simulink library "tenneco_lib"  (R2016b)
settings: Solver=ode45  StartTime=0.0  StopTime=10.0  RelTol=1e-3
undefined symbols (not defined in the file): Com_cntAMBInitTO_c, Com_cntAMBStopTO_c, Com_cntEC1InitTO_c, Com_cntEC1StopTO_c, Com_swAMBRx_c, Com_swEC1Rx_c, Com_swUseSPN108_c, Com_swUseSPN543_c, const, Env_pAmbPDflt_c, Env_pAmbPKOff_c, Env_pAmbPOvrd_c, Env_swAmbPOvrd_c, MSG_INIT_TIMEOUT, MSG_NOT_RECEIVED, MSG_RECEIVED_NOW, MSG_STOP_TIMEOUT
libraries: simulink x19, tenneco_lib x2
(part 1 of 5)
settings Model: Creator=artimahe  LastModifiedBy=jwd5048
settings Model: ModifiedComment=|
  | jwd5048 -- Fri Dec 14 12:11:19 2018 -- Version 1.13
  | 
  | Changed Rate Trasnition block info to have output sample time visible; Updated SWC template to have root level I/O; Subsyetem librart blocks (filters, timers etc) are set to run as Atomic
settings Model: ModifiedHistory=|
  | jwd5048 -- Fri Dec 14 12:11:19 2018 -- Version 1.13
  | 
  | Changed Rate Trasnition block info to have output sample time visible; Updated SWC template to have root level I/O; Subsyetem librart blocks (filters, timers etc) are set to run as Atomic
  | 
  | jwd5048 -- Sun Dec 09 17:40:26 2018 -- Version 1.12
  | 
  | Added report generator inport, outport, documentation blocks, Report Generator Subsystem, Updated LUTs for output data type in table data
settings DataIOCC: LimitDataPoints=on  SaveFormat=Array
settings OptimizationCC: BlockReduction=off  BooleanDataType=off  LifeSpan=inf
settings DebuggingCC: SaveWithParameterizedLinksMsg=none  UnderspecifiedInitializationDetection=Classic  MergeDetectMultiDrivingBlocksExec=none  SignalResolutionControl=TryResolveAllWithWarning  StrictBusMsg=Warning  SFUnexpectedBacktrackingDiag=warning  SFNoUnconditionalDefaultTransitionDiag=warning  SFExecutionAtInitializationDiag=none
settings HardwareCC: ProdBitPerPointer=32  ProdBitPerSizeT=32  ProdBitPerPtrDiffT=32  ProdLargestAtomicFloat=None  ProdIntDivRoundTo=Undefined  ProdEndianess=Unspecified  ProdWordSize=32  ProdHWDeviceType=32-bit Generic  TargetUnknown=on
settings ModelReferenceCC: PropagateSignalLabelsOutOfModel=off
settings GRTTargetCC: TargetLangStandard=C89/C90 (ANSI)  GeneratePreprocessorConditionals=Disable all
settings ConfigComp: CovMetricSettings=dw  CovHtmlReporting=on  CovSaveCumulativeToWorkspaceVar=on  CovSaveSingleToWorkspaceVar=on  CovExternalEMLEnable=off  CovSFcnEnable=off

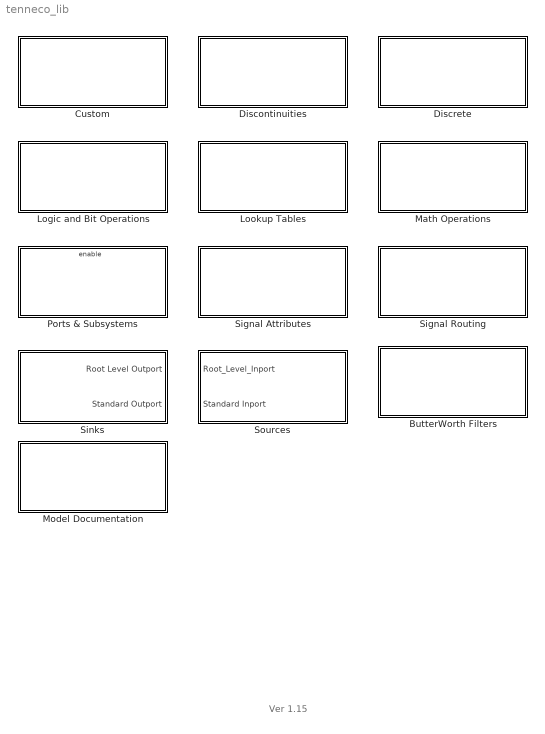
== system tenneco_lib ==
  note: Ver 1.15
  ButterWorth Filters : Subsystem
      mask Display: disp('Filters');
  Custom : Subsystem
      mask Display: disp('Custom');
  Discontinuities : Subsystem
      mask Display: disp('Discontinuities');
  Discrete : Subsystem
      mask Display: disp('Discrete');
  Logic and Bit Operations : Subsystem
      mask Display: disp('Logic and Bit Operations');
  Lookup Tables : Subsystem
      mask Display: disp('Lookup Tables');
  Math Operations : Subsystem
      mask Display: disp('Math Operations');
  Model Documentation : Subsystem
      mask Display: disp('Model Documentation');
  Ports & Subsystems : Subsystem
      mask Display: disp('Ports & Subsystems');
  Signal Attributes : Subsystem
      mask Display: disp('Signal Attributes');
  Signal Routing : Subsystem
      mask Display: disp('Signal Routing');
  Sinks : Subsystem
      mask Display: disp('Sinks');
  Sources : Subsystem
      mask Display: disp('Sources');

== system tenneco_lib/ButterWorth Filters ==
  Butterworth First Order HPF : Subsystem  TreatAsAtomicUnit=on  mask(Filter){Ts=.001}
      mask prompts: Ts "sample time(sec)"
      mask help: Butterworth First Order HPF
      mask Display:
      | image(imread('Tenneco_Copyright_Logo_Mini.bmp'),'center');
      | color('red');
      | disp('\n\n\n\n\n\n\nTenneco Confidential Red\n Restricted. Do not Distribute.');
  Butterworth First Order LPF : Subsystem  TreatAsAtomicUnit=on  mask(Filter){Ts=.001}
      mask prompts: Ts "sample time(sec)"
      mask help: Butterworth First Order LPF
      mask Display:
      | image(imread('Tenneco_Copyright_Logo_Mini.bmp'),'center');
      | color('red');
      | disp('\n\n\n\n\n\n\nTenneco Confidential Red\n Restricted. Do not Distribute.');
  Butterworth Second Order BPF : Subsystem  TreatAsAtomicUnit=on  mask(Filter){Ts=0.001}
      mask prompts: Ts "sample time(sec)"
      mask help: Butterworth Second Order BPF
      mask Display:
      | image(imread('Tenneco_Copyright_Logo_Mini.bmp'),'center');
      | color('red');
      | disp('\n\n\n\n\n\n\nTenneco Confidential Red\n Restricted. Do not Distribute.');
  Butterworth Second Order HPF : Subsystem  TreatAsAtomicUnit=on  mask(Filter){Ts=.001}
      mask prompts: Ts "sample time(sec)"
      mask help: Butterworth Second Order HPF
      mask Display:
      | image(imread('Tenneco_Copyright_Logo_Mini.bmp'),'center');
      | color('red');
      | disp('\n\n\n\n\n\n\nTenneco Confidential Red\n Restricted. Do not Distribute.');
  Butterworth Second Order LPF : Subsystem  TreatAsAtomicUnit=on  mask(Filter){Ts=.001}
      mask prompts: Ts "sample time(sec)"
      mask help: Butterworth Second Order LPF
      mask Display:
      | image(imread('Tenneco_Copyright_Logo_Mini.bmp'),'center');
      | color('red');
      | disp('\n\n\n\n\n\n\nTenneco Confidential Red\n Restricted. Do not Distribute.');
  Generic Low-Pass Filter : Subsystem  TreatAsAtomicUnit=on  mask{Fil=.01, SampleTime=1, N=2}
      mask prompts: Fil "Filter Coefficient"; SampleTime "Sample Time in Seconds"; N "Stabilization Time [# loops]"
      mask help:
      | Filter coefficient=sampletime/number of samples to be averaged
      | Please use explicit sample time. Do not use (-1).
      |
      | The initial condition of the filter will be the input value after the
      | stabilization period has expired.
      mask Display:
      | port_label('input',1,'x');
      | port_label('output',1,'y');
      | 
      | image(imread('Tenneco_Copyright_Logo_Mini.bmp'),'center');
      | color('red');
      | disp('\n\n\n\n\n\n\nTenneco Confidential Red\n Restricted. Do not Distribute.');
  Resettable Variable Low-Pass Filter : Subsystem  TreatAsAtomicUnit=on  mask{Ts=0.1, N=2}
      mask prompts: Ts "Filter Sample Time [sec]"; N "Stabilization Loops [#]"
      mask help:
      | The initial condition of the filter will be the input value after the
      | stabilization period has expired.
      mask init:
      | if (isempty(N) || ...
      |         rem(N, 1) ~= 0 || ...
      |        (rem(N, 1) == 0 && N < 1))
      |         errordlg(['Number of stabilization loops must be a ' ...
      |                  'positive integer.'], ...
      |                  'Error: Function Block Parameters');
      | end
      | 
      | if (isempty(Ts) || ...
      |         (Ts <= 0))
      |         errordlg(['Sample time must be greater than zero.'], ...
      |                  'Error: Function Block Parameters');
      | end
      mask Display:
      | port_label('input',1,'x');
      | port_label('input',2,'t [sec]');
      | port_label('input',3,'reset');
      | port_label('output',1,'y');
      | 
      | image(imread('Tenneco_Copyright_Logo_Mini.bmp'),'center');
      | color('red');
      | disp('\n\n\n\n\n\n\nTenneco Confidential Red\n Restricted. Do not Distribute.');
  Variable Low-Pass Filter : Subsystem  TreatAsAtomicUnit=on  mask{Ts=0.1, N=2}
      mask prompts: Ts "Filter Sample Time [sec]"; N "Stabilization Loops [#]"
      mask help:
      | The initial condition of the filter will be the input value after the
      | stabilization period has expired.
      mask init: same as tenneco_lib/ButterWorth Filters/Resettable Variable Low-Pass Filter
      mask Display:
      | port_label('input',1,'x');
      | port_label('input',2,'\tau [sec]','texmode','on');
      | port_label('output',1,'y');
      | 
      | image(imread('Tenneco_Copyright_Logo_Mini.bmp'),'center');
      | color('red');
      | disp('\n\n\n\n\n\n\nTenneco Confidential Red\n Restricted. Do not Distribute.');

== system tenneco_lib/Custom ==
  CAN : Subsystem
      mask Display: disp('CAN');
  Logical : Subsystem
      mask Display: disp('Logical');
  Math : Subsystem
      mask Display: disp('Math');
  Timers : Subsystem
      mask Display: disp('Timers');

== system tenneco_lib/Discontinuities ==
  Rate Limiter Dynamic : simulink/Discontinuities/Rate Limiter Dynamic
  Saturation : Saturate  UpperLimit=UpperLimit  LowerLimit=LowerLimit  mask(Saturation){UpperLimit=0.5, LowerLimit=-0.5}
      mask prompts: UpperLimit "Simulink:blkprm_prompts:SaturateUpLim"; LowerLimit "Simulink:blkprm_prompts:SaturateLowLim"
      mask help: Limit input signal to the upper and lower saturation values.
      settings: CopyFcn=set_param(gcbh,'LinkStatus','none');
      mask TypeOptions UpperLimit: UpperLimit
      mask TypeOptions LowerLimit: LowerLimit

== system tenneco_lib/Discrete ==
  Discrete Filter : DiscreteFilter  NumeratorSource=Input port  DenominatorSource=Input port  a0EqualsOne=on  mask(Discrete Filter){}
      mask help: Independently filter each channel of the input over time using a discrete IIR filter. Specify the numerator and denominator coefficients in ascending order of powers of 1/z.
      settings: CopyFcn=set_param(gcbh,'LinkStatus','none');  InputPortMap=u0,p1,p3
  Unit Delay : UnitDelay  InitialCondition=InitialCondition  SampleTime=-1  mask(Unit Delay){InitialCondition=0}
      mask prompts: InitialCondition "Simulink:blkprm_prompts:DelayBlkInitCond"
      mask help: Sample and hold with one sample period delay.
      settings: CopyFcn=set_param(gcbh,'LinkStatus','none');
      mask TypeOptions InitialCondition: InitialCondition

== system tenneco_lib/Logic and Bit Operations ==
  Bitwise Operator : simulink/Logic and Bit Operations/Bitwise Operator  logicop=AND  UseBitMask=on  BitMask=bin2dec('11011001')  BitMaskRealWorld=Stored Integer
  Compare To Constant : simulink/Logic and Bit Operations/Compare To Constant  relop=<=  const=const  OutDataTypeStr=boolean
  Logical Operator : Logic  Inputs=Inputs  AllPortsSameDT=off  OutDataTypeStr=boolean  mask(Logical Operator){Operator=AND, Inputs=2}
      mask prompts: Operator "Simulink:blkprm_prompts:LogicOperator"; Inputs "Simulink:blkprm_prompts:LogicNumInputPorts"
      mask help: Logical operators. For a single input, operators are applied across the input vector. For multiple inputs, operators are applied across the inputs.
      settings: CopyFcn=set_param(gcbh,'LinkStatus','none');
      mask TypeOptions Operator: Operator
      mask TypeOptions Inputs: Inputs
  Relational Operator : RelationalOperator  Operator=<=  OutDataTypeStr=boolean  RndMeth=Nearest  mask(Relational Operator){Operator=<=}
      mask prompts: Operator "Simulink:blkprm_prompts:RelopOperator"
      mask help: Applies the selected relational operator to the inputs and outputs the result. The top (or left) input corresponds to the first operand.
      settings: CopyFcn=set_param(gcbh,'LinkStatus','none');
      mask TypeOptions Operator: Operator
  Shift Arithmetic : ArithShift  BitShiftNumber=8
      settings: CopyFcn=set_param(gcbh,'LinkStatus','none');

== system tenneco_lib/Lookup Tables ==
  1-D Lookup Table : Lookup_n-D  NumberOfTableDimensions=1  BreakpointsForDimension1=BreakpointsForDimension1  BreakpointsForDimension3=[5, 7]  Table=Table  ExtrapMethod=Clip  UseLastTableValue=on  InternalRulePriority=Speed  OutDataTypeStr=Inherit: Inherit from 'Table data'  RndMeth=Simplest  LockScale=on  mask(Lookup Table (1-D)){Table=[1,2,3], BreakpointsForDimension1=[10,22,31]}
      mask prompts: Table "Simulink:blkprm_prompts:InterpndTable"; BreakpointsForDimension1 "Breakpoints for axis:"
      mask help: Perform 1-dimensional interpolated table lookup including index searches. The table is a sampled representation of a function in N variables. Breakpoint sets relate the input values to positions in the table.
      settings: CopyFcn=set_param(gcbh,'LinkStatus','none');
      mask TypeOptions Table: Table
      mask TypeOptions BreakpointsForDimension1: BreakpointsForDimension1
  2-D Lookup Table : Lookup_n-D  BreakpointsForDimension1=BreakpointsForDimension1  BreakpointsForDimension2=BreakpointsForDimension2  BreakpointsForDimension3=[5, 7]  Table=Table  ExtrapMethod=Clip  UseLastTableValue=on  InternalRulePriority=Speed  OutDataTypeStr=Inherit: Inherit from 'Table data'  RndMeth=Simplest  LockScale=on  mask(Lookup Table (2-D)){Table=[1,2,3;4,5,6], BreakpointsForDimension1=[10,22], BreakpointsForDimension2=[10,22,31]}
      mask prompts: Table "Simulink:blkprm_prompts:InterpndTable"; BreakpointsForDimension1 "Breakpoints for u1 (y-axis):"; BreakpointsForDimension2 "Breakpoints for u2 (x-axis):"
      mask help: Perform 2-dimensional interpolated table lookup including index searches. The table is a sampled representation of a function in N variables. Breakpoint sets relate the input values to positions in the table. The first dimension corresponds to the top (or left) input port.
      settings: CopyFcn=set_param(gcbh,'LinkStatus','none');
      mask TypeOptions Table: Table
      mask TypeOptions BreakpointsForDimension1: BreakpointsForDimension1
      mask TypeOptions BreakpointsForDimension2: BreakpointsForDimension2

== system tenneco_lib/Math Operations ==
  Abs : Abs  mask(Abs){}
      mask help: y = |u|
      settings: CopyFcn=set_param(gcbh,'LinkStatus','none');
  Gain : Gain  Gain=Gain  mask(Gain){Gain=1}
      mask prompts: Gain "Simulink:blkprm_prompts:GainGain"
      mask help: Element-wise gain (y = K.*u) or matrix gain (y = K*u or y = u*K).
      mask init:
      | blkName = gcb;
      | 
      | str = ['C']; %default
      | 
      | const_str = get_param(blkName, 'Gain');
      | const_val = str2num(const_str);
      | 
      | if isempty(const_val) %#ok<ST2NM>
      |     %Expression/Variable
      |     str = [strtrim(const_str)];
      | else
      |     if length(const_val) == 1 
      |         if Simulink.data.isSupportedEnumClass(class(const_val))
      |             % Special Handling for Enumerations
      |             if Simulink.data.getEnumTypeInfo(class(const_val), 'AddClassNameToEnumNames')
      |                 str = [strtrim(const_str)];
      |             else
      |                 str = [char(const_val)];
      |             end
      |         elseif(isfloat(const_val) || isinteger(const_val)) 
      |                 str = [num2str(const_val)];
      |         end
      |     end
      | end
      settings: CopyFcn=set_param(gcbh,'LinkStatus','none');
      mask TypeOptions Gain: Gain
      mask Display: disp(strcat('GAIN\n',str))
  Math Function : Math  Operator=square  SaturateOnIntegerOverflow=on  mask(Math){Operator=square}
      mask prompts: Operator "SimulinkBlocks:dialog:BmathfcnOperator"
      mask help: Mathematical functions including logarithmic, exponential, power, and modulus functions. When the function has more than one argument, the first argument corresponds to the top (or left) input port.
      settings: CopyFcn=set_param(gcbh,'LinkStatus','none');
      mask TypeOptions Operator: Operator
  MinMax : MinMax  Inputs=Inputs  mask(MinMax){Function=min, Inputs=1}
      mask prompts: Function "Simulink:blkprm_prompts:MinMaxFunction"; Inputs "Simulink:blkprm_prompts:MinMaxNumInPorts"
      mask help: Output min or max of input. For a single input, operators are applied across the input vector. For multiple inputs, operators are applied across the inputs.
      settings: CopyFcn=set_param(gcbh,'LinkStatus','none');
      mask TypeOptions Function: Function
      mask TypeOptions Inputs: Inputs
  Product : Product  Inputs=*/  InputSameDT=on  mask(Product){Inputs=*/}
      mask prompts: Inputs "List of signs:"
      mask help:
      | Multiply or divide inputs.  Specify one of the following:
      |  a) * or / for each input port. For example, **/* performs the operation 'u1*u2/u3*u4'.
      |  b) scalar specifies the number of input ports to be multiplied.
      settings: CopyFcn=set_param(gcbh,'LinkStatus','none');
      mask TypeOptions Inputs: Inputs
  Rounding Function : Rounding  Operator=round  mask(Rounding){Operator=round}
      mask prompts: Operator "Simulink:blkprm_prompts:RoundOperator"
      mask help: Rounding operations.
      settings: CopyFcn=set_param(gcbh,'LinkStatus','none');
      mask TypeOptions Operator: Operator
  Sqrt : Sqrt  SaturateOnIntegerOverflow=on  mask(Sqrt){Operator=sqrt}
      mask prompts: Operator "SimulinkBlocks:SqrtFcn:BmathfcnOperator"
      mask help: Square root functions including square root, signed square root, and reciprocal square root functions.
      settings: CopyFcn=set_param(gcbh,'LinkStatus','none');
      mask TypeOptions Operator: Operator
  Sum : Sum  Inputs=+-  InputSameDT=on  mask(Sum){Inputs=+-}
      mask prompts: Inputs "Simulink:blkprm_prompts:SumListofSigns"
      mask help:
      | Add or subtract inputs.  Specify one of the following:
      | a) character vector containing + or - for each input port, | for spacer between ports (e.g. ++|-|++)
      | b) scalar, >= 1, specifies the number of input ports to be summed.
      | When there is only one input port, add or subtract elements over all dimensions or one specified dimension
      settings: CopyFcn=set_param(gcbh,'LinkStatus','none');
      mask TypeOptions Inputs: Inputs
  Trigonometric Function : Trigonometry  mask(Trigonometric Function){Operator=sin}
      mask prompts: Operator "Simulink:blkprm_prompts:TrigFcnOperator"
      mask help: Trigonometric and hyperbolic functions. When the function has more than one argument, the first argument corresponds to the top (or left) input port.
      settings: CopyFcn=set_param(gcbh,'LinkStatus','none');
      mask TypeOptions Operator: Operator
  Unary Minus : UnaryMinus
      settings: CopyFcn=set_param(gcbh,'LinkStatus','none');

== system tenneco_lib/Model Documentation ==
  Appendix Title : Subsystem  mask(RptGen Appendix){rptgenOrder=10}
      mask prompts: rptgenOrder "Report Gen Order Priority"
      mask help:
      | This block is designed to contain RptGen Description and RptGen Detail blocks to create a document structure as an appendix to be added at the end of the MBDD.
      |
      | If this block is anywhere in a model, an appendix with the block name as the section title shall appear in the report.
      |
      | The Report Gen Order Priority allows the user to set the sorted order of the block's contents appearing in the report.
      settings: OpenFcn=open_system(gcb,'force')
      mask Display: disp(['Appendix - ',get_param(gcb,'rptgenOrder')])
  Description : Subsystem  mask(RptGenDescription){rptgenOrder=10}
      mask prompts: rptgenOrder "Report Gen Order Priority"
      mask help:
      | This block can contain text, tables, lists, images, and equations from a Word document to describe its parent subsystem.
      |
      | The contents of this block shall be placed in paragraph(s) just after the subsystem's section heading in the report, before the system snapshot.
      |
      | The Report Gen Order Priority allows the user to set the sorted order of the block's contents appearing in the report.
      settings: OpenFcn=open_system([gcb,'/DocBlock'])
      mask Display: disp(['Description - ',get_param(gcb,'rptgenOrder')])
  Detail : Subsystem  mask(RptGenDetail){rptgenOrder=10}
      mask prompts: rptgenOrder "Report Gen Order Priority"
      mask help:
      | This block can contain text, tables, lists, images, and equations from a Word document to further describe its parent subsystem, when a brief description is not sufficient to fully describe a system.
      |
      | The name of this block shall appear as the subsection title underneath the current subsystem's section.
      |
      | The Report Gen Order Priority allows the user to set the sorted order of the block's contents appearing in the report.
      settings: OpenFcn=open_system([gcb,'/DocBlock'])
      mask Display: disp(['Detail - ',get_param(gcb,'rptgenOrder')])
  Introduction : Subsystem  mask(RptGenIntroduction){rptgenOrder=10}
      mask prompts: rptgenOrder "Report Gen Order Priority"
      mask help:
      | This block can contain text, tables, lists, images, and equations from a Word document for the introduction portion of the MBDD.
      |
      | The contents of this block shall be placed in the introductory section if it is in a software part model.
      |
      | The Report Gen Order Priority allows the user to set the sorted order of the block's contents appearing in the report.
      settings: OpenFcn=open_system([gcb,'/DocBlock'])
      mask Display: disp(['Introduction - ',get_param(gcb,'rptgenOrder')])

== system tenneco_lib/Ports & Subsystems ==
  Enable : EnablePort  mask(Enable Port){StatesWhenEnabling=held, ShowOutputPort=off}
      mask prompts: StatesWhenEnabling "Simulink:blkprm_prompts:EnabPortStates"; ShowOutputPort "Simulink:blkprm_prompts:TrigEnabShowOutPort"
      mask help: Place this block in a subsystem or at the root level of a model to create an enabled system.
      settings: CopyFcn=set_param(gcbh,'LinkStatus','none');
      mask TypeOptions StatesWhenEnabling: StatesWhenEnabling
      mask TypeOptions ShowOutputPort: ShowOutputPort
  If : If  mask(If Block){NumInputs=1, IfExpression=u1 > 0, ElseIfExpressions=, ShowElse=on}
      mask prompts: NumInputs "Simulink:blkprm_prompts:IfNumInputs"; IfExpression "Simulink:blkprm_prompts:IfCondition"; ElseIfExpressions "Simulink:blkprm_prompts:ElseIfConds"; ShowElse "Simulink:blkprm_prompts:IfShowElse"
      mask help:
      | IF expression
      |     Run the Action Subsystem connected to 1st output port
      | ELSEIF expression
      |     Run the Action Subsystem connected to 2nd output port
      | ELSE
      |     Run the Action Subsystem connected to last output port
      | END
      | The number of Elseif output ports in the block is equal to the
      | number of comma-separated Elseif expressions entered in the dialog.
      | The If and Elseif expressions can use these MATLAB operators:
      |     <, <=, ==, ~=, >, >=, &, |, ~, (  ), unary-minus
      | on the input port signals named u1, u2, u3, etc.
      settings: CopyFcn=set_param(gcbh,'LinkStatus','none');
      mask TypeOptions NumInputs: NumInputs
      mask TypeOptions IfExpression: IfExpression
      mask TypeOptions ElseIfExpressions: ElseIfExpressions
      mask TypeOptions ShowElse: ShowElse
  If Action Subsystem : Subsystem  TreatAsAtomicUnit=on
      settings: CopyFcn=set_param(gcbh,'LinkStatus','none'); set_param(gcbh,'Mask','off'); set_param(gcbh,'MaskType',''); set_param(gcbh,'MaskDescription',''); set_param(gcbh,'OpenFcn',''); set_param(gcbh,'CopyFcn','')  OpenFcn=open_system(gcbh,'force')
  SoftwareComponent SWC : Subsystem  Tag=SoftwareComponent  mask(Software Component Subsystem){libVer=1.13, DataDictionary=SoftwareComponent_dd.m, swDescription=, logEntry=|}
      mask logEntry=|
      | jwd5048 -- Fri Dec 14 12:11:19 2018 -- Version 1.13
      |
      | Changed Rate Trasnition block info to have output sample time visible; Updated SWC template to have root level I/O; Subsyetem librart blocks (filters, timers etc) are set to run as Atomic
      mask prompts: libVer "Library Version"; DataDictionary "Data Dictionary File"; swDescription "Software Description"; logEntry "Version Log"
      mask help: Keeps track of the version of the software component and the corresponding data dictionary. Also contains an abstract description of the software component and the last version log entry.
      settings: PreSaveFcn=updateSwcParams  OpenFcn=open_system(gcb,'force')
      mask Help: If this subsystem resides inside the top layer of a Simulink diagram, changing the version number in the parameters pane will kick-off operations to update the model history and version number.  It will also run checks to make sure the log entry was updated and the version number was incremented properly, before pushing this information to the model parameters.
      mask DialogControl Control3 Prompt: Library Version:  %<libVer>
      mask DialogControl Container3 Prompt: Software Description
      mask DialogControl Control4 Prompt: %<swDescription>
      mask DialogControl Container4 Prompt: Version Log Entry
      mask DialogControl Control5 Prompt: %<logEntry>
      mask Display: disp(['Library Ver. ', get_param(gcb,'libVer'), '\nDD File: ', get_param(gcb,'DataDictionary')]);
  wires:
  If/1 -> If Action Subsystem/Action

== system tenneco_lib/Signal Attributes ==
  Data Type Conversion : DataTypeConversion  mask(Data Type Conversion){OutDataTypeStr=Inherit: Inherit via back propagation}
      mask prompts: OutDataTypeStr "Simulink:blkprm_prompts:OUTPUT_UNIFIEDDATATYPE"
      mask help: Convert the input to the data type and scaling of the output.
      settings: CopyFcn=set_param(gcbh,'LinkStatus','none');
      mask TypeOptions OutDataTypeStr: OutDataTypeStr
  Rate Transition : RateTransition
      settings: AttributesFormatString=%<OutPortSampleTime>  CopyFcn=set_param(gcbh,'LinkStatus','none');

== system tenneco_lib/Signal Routing ==
  Bus Creator : BusCreator  Inputs=2
      settings: CopyFcn=set_param(gcbh,'LinkStatus','none');
  Bus Selector : BusSelector  OutputSignals=signal1,signal2
      settings: CopyFcn=set_param(gcbh,'LinkStatus','none');
  Data Store Memory : DataStoreMemory  ReadBeforeWriteMsg=warning  WriteAfterWriteMsg=warning  WriteAfterReadMsg=warning  InitialValue=InitialValue  ShowAdditionalParam=off  mask(Data Store Memory){DataStoreName=A, InitialValue=0, OutDataTypeStr=Inherit: auto, Dimensions=-1}
      mask prompts: DataStoreName "Simulink:blkprm_prompts:DstoreMemDstoreName"; InitialValue "Simulink:blkprm_prompts:DstoreMemInitvalue"; OutDataTypeStr "Simulink:blkprm_prompts:UNIFIEDDATATYPE"; Dimensions "Simulink:blkprm_prompts:DstoreMemDimensions"
      mask help: Define a memory region for use by the Data Store Read and Data Store Write blocks. All Read and Write blocks that are in the current (sub)system level or below and have the same data store name will be able to read from or write to this block.
      settings: CopyFcn=set_param(gcbh,'LinkStatus','none');
      mask TypeOptions DataStoreName: DataStoreName
      mask TypeOptions InitialValue: InitialValue
      mask TypeOptions OutDataTypeStr: OutDataTypeStr
      mask TypeOptions Dimensions: Dimensions
  Data Store Read : DataStoreRead  SampleTime=SampleTime  mask(Data Store Read){DataStoreName=A, SampleTime=-1}
      mask prompts: DataStoreName "Simulink:blkprm_prompts:DstoreMemDstoreName"; SampleTime "Simulink:blkprm_prompts:AllSrcBlksSampleTime"
      mask help: Read values from the specified data store.
      settings: CopyFcn=set_param(gcbh,'LinkStatus','none');
      mask TypeOptions DataStoreName: DataStoreName
      mask TypeOptions SampleTime: SampleTime
  Data Store Write : DataStoreWrite  mask(Data Store Write){DataStoreName=A}
      mask prompts: DataStoreName "Simulink:blkprm_prompts:DstoreMemDstoreName"
      mask help: Write values to the specified data store.
      settings: CopyFcn=set_param(gcbh,'LinkStatus','none');
      mask TypeOptions DataStoreName: DataStoreName
  Demux : Demux  Outputs=2  mask(Demux){Outputs=2}
      mask prompts: Outputs "Simulink:blkprm_prompts:DemuxNumOfOutputs"
      mask help: Split vector signals into scalars or smaller vectors.
      settings: CopyFcn=set_param(gcbh,'LinkStatus','none');
      mask TypeOptions Outputs: Outputs
  Merge : Merge  Inputs=Inputs  InitialOutput=InitialOutput  mask(Merge){Inputs=2, InitialOutput=[]}
      mask prompts: Inputs "Simulink:blkprm_prompts:MergeNumInputs"; InitialOutput "Simulink:blkprm_prompts:MergeInitOutput"
      mask help: Merge the input signals into a single output signal whose initial value is specified by the 'Initial output' parameter. If 'Initial output' is empty, the Merge block outputs the initial output of one of its driving blocks.
      settings: CopyFcn=set_param(gcbh,'LinkStatus','none');
      mask TypeOptions Inputs: Inputs
      mask TypeOptions InitialOutput: InitialOutput
  Multiport Switch : MultiPortSwitch  DataPortOrder=Specify indices  DataPortIndices=DataPortIndices  DiagnosticForDefault=Warning  mask(Multiport Switch){DataPortIndices={1,2,3}}
      mask prompts: DataPortIndices "Simulink:blkprm_prompts:MpSwitch_DataPortIndices"
      mask help: Pass through the input signals corresponding to the truncated value of the first input. The inputs are numbered top to bottom (or left to right). The first input port is the control port. The other input ports are data ports.
      settings: CopyFcn=set_param(gcbh,'LinkStatus','none');
      mask TypeOptions DataPortIndices: DataPortIndices
  Mux : Mux  Inputs=2  mask(Mux){Inputs=2}
      mask prompts: Inputs "Simulink:blkprm_prompts:MuxNumInputs"
      mask help: Multiplex scalar or vector signals.
      settings: CopyFcn=set_param(gcbh,'LinkStatus','none');
      mask TypeOptions Inputs: Inputs
  Selector : Selector  IndexMode=Zero-based  InputPortWidth=3  IndexOptions=Index vector (dialog)  Indices=[1]  OutputSizes=1
      settings: CopyFcn=set_param(gcbh,'LinkStatus','none');
  Switch : Switch  Threshold=0.5  mask(Switch){}
      mask help: Pass through input 1 when input 2 satisfies the selected criterion; otherwise, pass through input 3. The inputs are numbered top to bottom (or left to right). The first and third input ports are data ports, and the second input port is the control port. The criteria for control port 2 are u2 >= Threshold (0.5).
      settings: CopyFcn=set_param(gcbh,'LinkStatus','none');
  Vector Concatenate : Concatenate  NumInputs=NumInputs  mask(Concatenate){NumInputs=2}
      mask prompts: NumInputs "Simulink:blkprm_prompts:ConcatNumInputs"
      mask help:
      | Concatenate input signals of the same data type to create a contiguous output signal.
      |
      | In vector mode, all input signals must be either vectors or one-row [1xM] matrices or one-column [Mx1] matrices or a combination of vectors and either one-row matrices or one-column matrices. The output is a vector if all inputs are vectors. The output is a one-row or one-column matrix if any of the inputs are one-row or one-column matrices, respectively.
      settings: CopyFcn=set_param(gcbh,'LinkStatus','none');
      mask TypeOptions NumInputs: NumInputs

== system tenneco_lib/Sinks ==
  Terminator : Terminator
      settings: CopyFcn=set_param(gcbh,'LinkStatus','none');
  Root Level Outport : Outport  OutMin=OutMin  OutMax=OutMax  SampleTime=SampleTime  mask(Root Level Outport){Port=1, OutDataTypeStr=Inherit: auto, PortDimensions=-1, SampleTime=-1, OutMin=[], OutMax=[], Unit=inherit}
      mask prompts: Port "Simulink:blkprm_prompts:InOutportPortNum"; OutDataTypeStr "Simulink:blkprm_prompts:UNIFIEDDATATYPE"; PortDimensions "Simulink:blkprm_prompts:InportPortDims"; SampleTime "Simulink:blkprm_prompts:AllBlksSampleTime"; OutMin "Simulink:blkprm_prompts:DesignMin"; OutMax "Simulink:blkprm_prompts:DesignMax"; Unit "Simulink:blkprm_prompts:OutputUnit_EditField"
      mask help: Provide a root level output port for a model.
      settings: CopyFcn=set_param(gcbh,'LinkStatus','none');
      mask TypeOptions Port: Port
      mask TypeOptions OutDataTypeStr: OutDataTypeStr
      mask TypeOptions PortDimensions: PortDimensions
      mask TypeOptions SampleTime: SampleTime
      mask TypeOptions OutMin: OutMin
      mask TypeOptions OutMax: OutMax
      mask TypeOptions Unit: Unit
  Standard Outport : Outport  Port=2  mask(Standard Outport){Port=2}
      mask prompts: Port "Simulink:blkprm_prompts:InOutportPortNum"
      mask help: Provide an output port for subsystems.
      settings: CopyFcn=set_param(gcbh,'LinkStatus','none');
      mask TypeOptions Port: Port

== system tenneco_lib/Sources ==
  Root_Level_Inport : Inport  OutMin=OutMin  OutMax=OutMax  Unit=m/s  PortDimensions=1  SampleTime=SampleTime  mask(Root Level Inport){Port=1, OutDataTypeStr=Inherit: auto, PortDimensions=1, Resolution=0.001, OutMin=-10, OutMax=10, Unit=m/s, SampleTime=-1, varSource=SoftwarePart_dd}
      mask prompts: Port "Simulink:blkprm_prompts:InOutportPortNum"; OutDataTypeStr "Simulink:blkprm_prompts:UNIFIEDDATATYPE"; PortDimensions "Simulink:blkprm_prompts:InportPortDims"; OutMin "Simulink:blkprm_prompts:DesignMin"; OutMax "Simulink:blkprm_prompts:DesignMax"; Unit "Simulink:blkprm_prompts:OutputUnit_EditField"; SampleTime "Simulink:blkprm_prompts:AllBlksSampleTime"; varSource "Signal Source"
      mask help:
      | Provide an input port for a software component.
      |
      | The data type, dimensions, and engineering units should be defined to detect mismatched properties to connected signals, and for design document generatioin.
      |
      | Minimum, maximum, and source should be filled in for report generation.
      settings: AttributesFormatString=%<Unit>  CopyFcn=set_param(gcbh,'LinkStatus','none');
      mask TypeOptions Port: Port
      mask TypeOptions OutDataTypeStr: OutDataTypeStr
      mask TypeOptions PortDimensions: PortDimensions
      mask TypeOptions OutMin: OutMin
      mask TypeOptions OutMax: OutMax
      mask TypeOptions Unit: Unit
      mask TypeOptions SampleTime: SampleTime
  Standard Inport : Inport  Port=2  mask(Standard Inport){Port=2}
      mask prompts: Port "Simulink:blkprm_prompts:InOutportPortNum"
      mask help: Provide an input port for subsystems.
      settings: CopyFcn=set_param(gcbh,'LinkStatus','none');
      mask TypeOptions Port: Port
  Constant : Constant  Value=Value  mask(Constant){Value=1}
      mask prompts: Value "Simulink:blkprm_prompts:ConstConstValue"
      mask help: Output the constant specified by the 'Constant value' parameter. If 'Constant value' is a vector, treat the constant value as a 1-D array.
      mask init:
      | blkName = gcb;
      | 
      | str = ['C']; %default
      | 
      | const_str = get_param(blkName, 'Value');
      | const_val = str2num(const_str);
      | 
      | if isempty(const_val) %#ok<ST2NM>
      |     %Expression/Variable
      |     str = [strtrim(const_str)];
      | else
      |     if length(const_val) == 1 
      |         if Simulink.data.isSupportedEnumClass(class(const_val))
      |             % Special Handling for Enumerations
      |             if Simulink.data.getEnumTypeInfo(class(const_val), 'AddClassNameToEnumNames')
      |                 str = [strtrim(const_str)];
      |             else
      |                 str = [char(const_val)];
      |             end
      |         elseif(isfloat(const_val) || isinteger(const_val) || islogical(const_val)) 
      |                 str = [num2str(const_val)];
      |         end
      |     end
      | end
      settings: CopyFcn=set_param(gcbh,'LinkStatus','none');
      mask TypeOptions Value: Value
      mask Display: disp(str)
  Ground : Ground  mask(Ground){}
      mask help: Used to "ground" input signals. (Prevents warnings about unconnected input ports.) Outputs zero.
      settings: CopyFcn=set_param(gcbh,'LinkStatus','none');

== system tenneco_lib/ButterWorth Filters/Butterworth First Order HPF ==
  x : Inport  mask(Standard Inport){Port=1}
      mask prompts: Port "Simulink:blkprm_prompts:InOutportPortNum"
      mask help: Provide an input port for subsystems.
      mask TypeOptions Port: Port
  CutOffFreq : Inport  Port=2  mask(Standard Inport){Port=2}
      mask prompts: Port "Simulink:blkprm_prompts:InOutportPortNum"
      mask help: Provide an input port for subsystems.
      mask TypeOptions Port: Port
  Coefficient Calculation : Subsystem
  Product1 : Product  Inputs=**  InputSameDT=on  mask(Product){Inputs=**}
      mask prompts: Inputs "List of signs:"
      mask help:
      | Multiply or divide inputs.  Specify one of the following:
      |  a) * or / for each input port. For example, **/* performs the operation 'u1*u2/u3*u4'.
      |  b) scalar specifies the number of input ports to be multiplied.
      mask TypeOptions Inputs: Inputs
  Product3 : Product  Inputs=**  InputSameDT=on  mask(Product){Inputs=**}
      mask prompts: Inputs "List of signs:"
      mask help:
      | Multiply or divide inputs.  Specify one of the following:
      |  a) * or / for each input port. For example, **/* performs the operation 'u1*u2/u3*u4'.
      |  b) scalar specifies the number of input ports to be multiplied.
      mask TypeOptions Inputs: Inputs
  Product4 : Product  Inputs=**  InputSameDT=on  mask(Product){Inputs=**}
      mask prompts: Inputs "List of signs:"
      mask help:
      | Multiply or divide inputs.  Specify one of the following:
      |  a) * or / for each input port. For example, **/* performs the operation 'u1*u2/u3*u4'.
      |  b) scalar specifies the number of input ports to be multiplied.
      mask TypeOptions Inputs: Inputs
  Sum1 : Sum  InputSameDT=on  mask(Sum){Inputs=++}
      mask prompts: Inputs "Simulink:blkprm_prompts:SumListofSigns"
      mask help:
      | Add or subtract inputs.  Specify one of the following:
      | a) character vector containing + or - for each input port, | for spacer between ports (e.g. ++|-|++)
      | b) scalar, >= 1, specifies the number of input ports to be summed.
      | When there is only one input port, add or subtract elements over all dimensions or one specified dimension
      mask TypeOptions Inputs: Inputs
  Sum2 : Sum  Inputs=+-  InputSameDT=on  mask(Sum){Inputs=+-}
      mask prompts: Inputs "Simulink:blkprm_prompts:SumListofSigns"
      mask help:
      | Add or subtract inputs.  Specify one of the following:
      | a) character vector containing + or - for each input port, | for spacer between ports (e.g. ++|-|++)
      | b) scalar, >= 1, specifies the number of input ports to be summed.
      | When there is only one input port, add or subtract elements over all dimensions or one specified dimension
      mask TypeOptions Inputs: Inputs
  Unit Delay1 : UnitDelay  InitialCondition=InitialCondition  SampleTime=-1  mask(Unit Delay){InitialCondition=0}
      mask prompts: InitialCondition "Simulink:blkprm_prompts:DelayBlkInitCond"
      mask help: Sample and hold with one sample period delay.
      mask TypeOptions InitialCondition: InitialCondition
  Unit Delay2 : UnitDelay  InitialCondition=InitialCondition  SampleTime=-1  mask(Unit Delay){InitialCondition=0}
      mask prompts: InitialCondition "Simulink:blkprm_prompts:DelayBlkInitCond"
      mask help: Sample and hold with one sample period delay.
      mask TypeOptions InitialCondition: InitialCondition
  y : Outport  mask(Standard Outport){Port=1}
      mask prompts: Port "Simulink:blkprm_prompts:InOutportPortNum"
      mask help: Provide an output port for subsystems.
      mask TypeOptions Port: Port
  wires:
  CutOffFreq/1 -> Coefficient Calculation/1(CutOffFreq)
  Sum1/1 -> y/1, Unit Delay2/1
  Unit Delay2/1 -> Product4/1
  [a0] -> Product4/2
  Product4/1 -> Sum2/2
  Sum2/1 -> Sum1/2
  Product1/1 -> Sum2/1
  [b1] -> Product1/1
  Unit Delay1/1 -> Product1/2
  Product3/1 -> Sum1/1
  Coefficient Calculation/2(b0) -> [b0]
  Coefficient Calculation/3(b1) -> [b1]
  Coefficient Calculation/1(a0) -> [a0]
  x/1 -> Product3/1, Unit Delay1/1
  [b0] -> Product3/2

== system tenneco_lib/ButterWorth Filters/Butterworth First Order LPF ==
  x : Inport  mask(Standard Inport){Port=1}
      mask prompts: Port "Simulink:blkprm_prompts:InOutportPortNum"
      mask help: Provide an input port for subsystems.
      mask TypeOptions Port: Port
  CutOffFreq : Inport  Port=2  mask(Standard Inport){Port=2}
      mask prompts: Port "Simulink:blkprm_prompts:InOutportPortNum"
      mask help: Provide an input port for subsystems.
      mask TypeOptions Port: Port
  Coefficient Calculation : Subsystem
  Product3 : Product  Inputs=**  InputSameDT=on  mask(Product){Inputs=**}
      mask prompts: Inputs "List of signs:"
      mask help:
      | Multiply or divide inputs.  Specify one of the following:
      |  a) * or / for each input port. For example, **/* performs the operation 'u1*u2/u3*u4'.
      |  b) scalar specifies the number of input ports to be multiplied.
      mask TypeOptions Inputs: Inputs
  Product4 : Product  Inputs=**  InputSameDT=on  mask(Product){Inputs=**}
      mask prompts: Inputs "List of signs:"
      mask help:
      | Multiply or divide inputs.  Specify one of the following:
      |  a) * or / for each input port. For example, **/* performs the operation 'u1*u2/u3*u4'.
      |  b) scalar specifies the number of input ports to be multiplied.
      mask TypeOptions Inputs: Inputs
  Product5 : Product  Inputs=**  InputSameDT=on  mask(Product){Inputs=**}
      mask prompts: Inputs "List of signs:"
      mask help:
      | Multiply or divide inputs.  Specify one of the following:
      |  a) * or / for each input port. For example, **/* performs the operation 'u1*u2/u3*u4'.
      |  b) scalar specifies the number of input ports to be multiplied.
      mask TypeOptions Inputs: Inputs
  Sum2 : Sum  InputSameDT=on  mask(Sum){Inputs=++}
      mask prompts: Inputs "Simulink:blkprm_prompts:SumListofSigns"
      mask help:
      | Add or subtract inputs.  Specify one of the following:
      | a) character vector containing + or - for each input port, | for spacer between ports (e.g. ++|-|++)
      | b) scalar, >= 1, specifies the number of input ports to be summed.
      | When there is only one input port, add or subtract elements over all dimensions or one specified dimension
      mask TypeOptions Inputs: Inputs
  Sum3 : Sum  Inputs=+-  InputSameDT=on  mask(Sum){Inputs=+-}
      mask prompts: Inputs "Simulink:blkprm_prompts:SumListofSigns"
      mask help:
      | Add or subtract inputs.  Specify one of the following:
      | a) character vector containing + or - for each input port, | for spacer between ports (e.g. ++|-|++)
      | b) scalar, >= 1, specifies the number of input ports to be summed.
      | When there is only one input port, add or subtract elements over all dimensions or one specified dimension
      mask TypeOptions Inputs: Inputs
  Unit Delay2 : UnitDelay  InitialCondition=InitialCondition  SampleTime=-1  mask(Unit Delay){InitialCondition=0}
      mask prompts: InitialCondition "Simulink:blkprm_prompts:DelayBlkInitCond"
      mask help: Sample and hold with one sample period delay.
      mask TypeOptions InitialCondition: InitialCondition
  Unit Delay3 : UnitDelay  InitialCondition=InitialCondition  SampleTime=-1  mask(Unit Delay){InitialCondition=0}
      mask prompts: InitialCondition "Simulink:blkprm_prompts:DelayBlkInitCond"
      mask help: Sample and hold with one sample period delay.
      mask TypeOptions InitialCondition: InitialCondition
  y : Outport  mask(Standard Outport){Port=1}
      mask prompts: Port "Simulink:blkprm_prompts:InOutportPortNum"
      mask help: Provide an output port for subsystems.
      mask TypeOptions Port: Port
  wires:
  Coefficient Calculation/1(a0) -> [a0]
  Coefficient Calculation/3(b1) -> [b1]
  Coefficient Calculation/2(b0) -> [b0]
  CutOffFreq/1 -> Coefficient Calculation/1(CutOffFreq)
  Sum2/1 -> y/1, Unit Delay3/1
  Unit Delay3/1 -> Product5/1
  [a0] -> Product5/2
  Product5/1 -> Sum3/2
  Sum3/1 -> Sum2/2
  Product3/1 -> Sum3/1
  [b1] -> Product3/1
  Unit Delay2/1 -> Product3/2
  Product4/1 -> Sum2/1
  x/1 -> Product4/1, Unit Delay2/1
  [b0] -> Product4/2

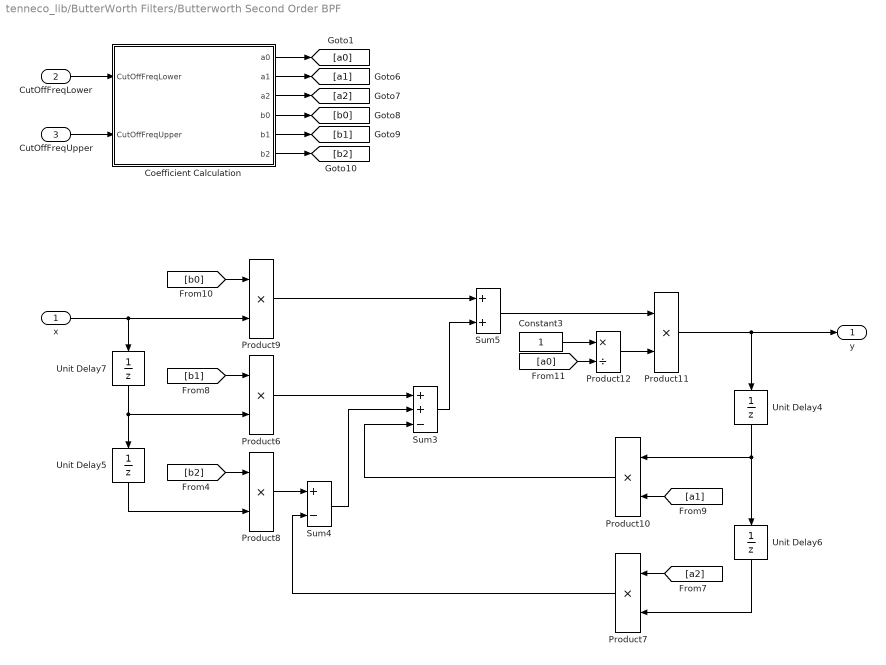
== system tenneco_lib/ButterWorth Filters/Butterworth Second Order BPF ==
  x : Inport  mask(Standard Inport){Port=1}
      mask prompts: Port "Simulink:blkprm_prompts:InOutportPortNum"
      mask help: Provide an input port for subsystems.
      mask TypeOptions Port: Port
  CutOffFreqLower : Inport  Port=2  mask(Standard Inport){Port=2}
      mask prompts: Port "Simulink:blkprm_prompts:InOutportPortNum"
      mask help: Provide an input port for subsystems.
      mask TypeOptions Port: Port
  CutOffFreqUpper : Inport  Port=3  mask(Standard Inport){Port=3}
      mask prompts: Port "Simulink:blkprm_prompts:InOutportPortNum"
      mask help: Provide an input port for subsystems.
      mask TypeOptions Port: Port
  Coefficient Calculation : Subsystem
  Constant3 : Constant  OutDataTypeStr=Inherit: Inherit via back propagation
  Product10 : Product  Inputs=**  InputSameDT=on  mask(Product){Inputs=**}
      mask prompts: Inputs "List of signs:"
      mask help:
      | Multiply or divide inputs.  Specify one of the following:
      |  a) * or / for each input port. For example, **/* performs the operation 'u1*u2/u3*u4'.
      |  b) scalar specifies the number of input ports to be multiplied.
      mask TypeOptions Inputs: Inputs
  Product11 : Product  Inputs=**  InputSameDT=on  mask(Product){Inputs=**}
      mask prompts: Inputs "List of signs:"
      mask help:
      | Multiply or divide inputs.  Specify one of the following:
      |  a) * or / for each input port. For example, **/* performs the operation 'u1*u2/u3*u4'.
      |  b) scalar specifies the number of input ports to be multiplied.
      mask TypeOptions Inputs: Inputs
  Product12 : Product  Inputs=*/  InputSameDT=on  mask(Product){Inputs=*/}
      mask prompts: Inputs "List of signs:"
      mask help:
      | Multiply or divide inputs.  Specify one of the following:
      |  a) * or / for each input port. For example, **/* performs the operation 'u1*u2/u3*u4'.
      |  b) scalar specifies the number of input ports to be multiplied.
      mask TypeOptions Inputs: Inputs
  Product6 : Product  Inputs=**  InputSameDT=on  mask(Product){Inputs=**}
      mask prompts: Inputs "List of signs:"
      mask help:
      | Multiply or divide inputs.  Specify one of the following:
      |  a) * or / for each input port. For example, **/* performs the operation 'u1*u2/u3*u4'.
      |  b) scalar specifies the number of input ports to be multiplied.
      mask TypeOptions Inputs: Inputs
  Product7 : Product  Inputs=**  InputSameDT=on  mask(Product){Inputs=**}
      mask prompts: Inputs "List of signs:"
      mask help:
      | Multiply or divide inputs.  Specify one of the following:
      |  a) * or / for each input port. For example, **/* performs the operation 'u1*u2/u3*u4'.
      |  b) scalar specifies the number of input ports to be multiplied.
      mask TypeOptions Inputs: Inputs
  Product8 : Product  Inputs=**  InputSameDT=on  mask(Product){Inputs=**}
      mask prompts: Inputs "List of signs:"
      mask help:
      | Multiply or divide inputs.  Specify one of the following:
      |  a) * or / for each input port. For example, **/* performs the operation 'u1*u2/u3*u4'.
      |  b) scalar specifies the number of input ports to be multiplied.
      mask TypeOptions Inputs: Inputs
  Product9 : Product  Inputs=**  InputSameDT=on  mask(Product){Inputs=**}
      mask prompts: Inputs "List of signs:"
      mask help:
      | Multiply or divide inputs.  Specify one of the following:
      |  a) * or / for each input port. For example, **/* performs the operation 'u1*u2/u3*u4'.
      |  b) scalar specifies the number of input ports to be multiplied.
      mask TypeOptions Inputs: Inputs
  Sum3 : Sum  Inputs=++-  InputSameDT=on  mask(Sum){Inputs=++-}
      mask prompts: Inputs "Simulink:blkprm_prompts:SumListofSigns"
      mask help:
      | Add or subtract inputs.  Specify one of the following:
      | a) character vector containing + or - for each input port, | for spacer between ports (e.g. ++|-|++)
      | b) scalar, >= 1, specifies the number of input ports to be summed.
      | When there is only one input port, add or subtract elements over all dimensions or one specified dimension
      mask TypeOptions Inputs: Inputs
  Sum4 : Sum  Inputs=+-  InputSameDT=on  mask(Sum){Inputs=+-}
      mask prompts: Inputs "Simulink:blkprm_prompts:SumListofSigns"
      mask help:
      | Add or subtract inputs.  Specify one of the following:
      | a) character vector containing + or - for each input port, | for spacer between ports (e.g. ++|-|++)
      | b) scalar, >= 1, specifies the number of input ports to be summed.
      | When there is only one input port, add or subtract elements over all dimensions or one specified dimension
      mask TypeOptions Inputs: Inputs
  Sum5 : Sum  InputSameDT=on  mask(Sum){Inputs=++}
      mask prompts: Inputs "Simulink:blkprm_prompts:SumListofSigns"
      mask help:
      | Add or subtract inputs.  Specify one of the following:
      | a) character vector containing + or - for each input port, | for spacer between ports (e.g. ++|-|++)
      | b) scalar, >= 1, specifies the number of input ports to be summed.
      | When there is only one input port, add or subtract elements over all dimensions or one specified dimension
      mask TypeOptions Inputs: Inputs
  Unit Delay4 : UnitDelay  InitialCondition=InitialCondition  SampleTime=-1  mask(Unit Delay){InitialCondition=0}
      mask prompts: InitialCondition "Simulink:blkprm_prompts:DelayBlkInitCond"
      mask help: Sample and hold with one sample period delay.
      mask TypeOptions InitialCondition: InitialCondition
  Unit Delay5 : UnitDelay  InitialCondition=InitialCondition  SampleTime=-1  mask(Unit Delay){InitialCondition=0}
      mask prompts: InitialCondition "Simulink:blkprm_prompts:DelayBlkInitCond"
      mask help: Sample and hold with one sample period delay.
      mask TypeOptions InitialCondition: InitialCondition
  Unit Delay6 : UnitDelay  InitialCondition=InitialCondition  SampleTime=-1  mask(Unit Delay){InitialCondition=0}
      mask prompts: InitialCondition "Simulink:blkprm_prompts:DelayBlkInitCond"
      mask help: Sample and hold with one sample period delay.
      mask TypeOptions InitialCondition: InitialCondition
  Unit Delay7 : UnitDelay  InitialCondition=InitialCondition  SampleTime=-1  mask(Unit Delay){InitialCondition=0}
      mask prompts: InitialCondition "Simulink:blkprm_prompts:DelayBlkInitCond"
      mask help: Sample and hold with one sample period delay.
      mask TypeOptions InitialCondition: InitialCondition
  y : Outport  mask(Standard Outport){Port=1}
      mask prompts: Port "Simulink:blkprm_prompts:InOutportPortNum"
      mask help: Provide an output port for subsystems.
      mask TypeOptions Port: Port
  wires:
  Coefficient Calculation/6(b2) -> [b2]
  Coefficient Calculation/3(a2) -> [a2]
  CutOffFreqLower/1 -> Coefficient Calculation/1(CutOffFreqLower)
  Coefficient Calculation/2(a1) -> [a1]
  Coefficient Calculation/5(b1) -> [b1]
  Coefficient Calculation/4(b0) -> [b0]
  CutOffFreqUpper/1 -> Coefficient Calculation/2(CutOffFreqUpper)
  Coefficient Calculation/1(a0) -> [a0]
  Unit Delay6/1 -> Product7/2
  Product7/1 -> Sum4/2
  [a2] -> Product7/1
  Sum4/1 -> Sum3/2
  Product8/1 -> Sum4/1
  Product10/1 -> Sum3/3
  Unit Delay5/1 -> Product8/2
  [b2] -> Product8/1
  x/1 -> Product9/2, Unit Delay7/1
  Product9/1 -> Sum5/1
  Unit Delay7/1 -> Unit Delay5/1, Product6/2
  [b1] -> Product6/1
  [b0] -> Product9/1
  Product6/1 -> Sum3/1
  Sum3/1 -> Sum5/2
  [a1] -> Product10/2
  Unit Delay4/1 -> Product10/1, Unit Delay6/1
  Sum5/1 -> Product11/1
  Product12/1 -> Product11/2
  [a0] -> Product12/2
  Constant3/1 -> Product12/1
  Product11/1 -> Unit Delay4/1, y/1
